simulink model "px4_direct_control"  (R2022b)
settings: Solver=FixedStepAuto  StartTime=0.0  StopTime=inf  RelTol=1e-3
undefined symbols (not defined in the file or in its folder): actuator, timestamp, timestamp_sample, xyz
libraries: ros2lib x8, aerolibutil x6, robotcorelib x1
settings Model: Creator=beniamino  LastModifiedBy=beniamino
settings OptimizationCC: EnhancedBackFolding=on  PassReuseOutputArgsAs=Individual arguments  ZeroExternalMemoryAtStartup=off  ZeroInternalMemoryAtStartup=off  MaxStackSize=64  OptimizeBlockOrder=speed  DifferentSizesBufferReuse=on  OptimizationCustomize=off  EfficientTunableParamExpr=on
settings DebuggingCC: ParameterTunabilityLossMsg=error
settings HardwareCC: ProdBitPerLong=64  ProdHWDeviceType=Intel->x86-64 (Linux 64)
settings SFSimCC: MATLABDynamicMemAlloc=off
settings RTWCC: Description=Embedded Coder  SystemTargetFile=ert.tlc  HardwareBoard=Robot Operating System 2 (ROS 2)  TLCOptions="-aInlineSetEventsForThisBaseRateFcn=TLC_FALSE -aSuppressMultiTaskScheduler=TLC_FALSE  -aRateBasedStepFcn=0"  TemplateMakefile=ert_default_tmf  Toolchain=Colcon Tools  TargetLang=C++
settings CodeAppCC: ForceParamTrailComments=on  IgnoreCustomStorageClasses=off  OperatorAnnotations=on  SimulinkDataObjDesc=on  SFDataObjDesc=on  InsertBlockDesc=on
settings ERTTargetCC: CodeInterfacePackaging=C++ class  RootIOFormat=Structure reference

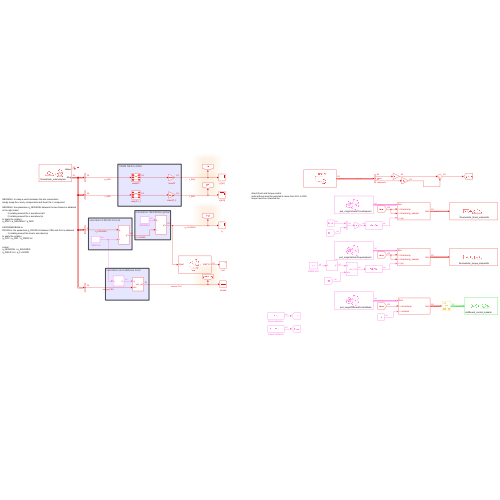
[thumbnail: Simulink's stored preview of the top-level diagram]
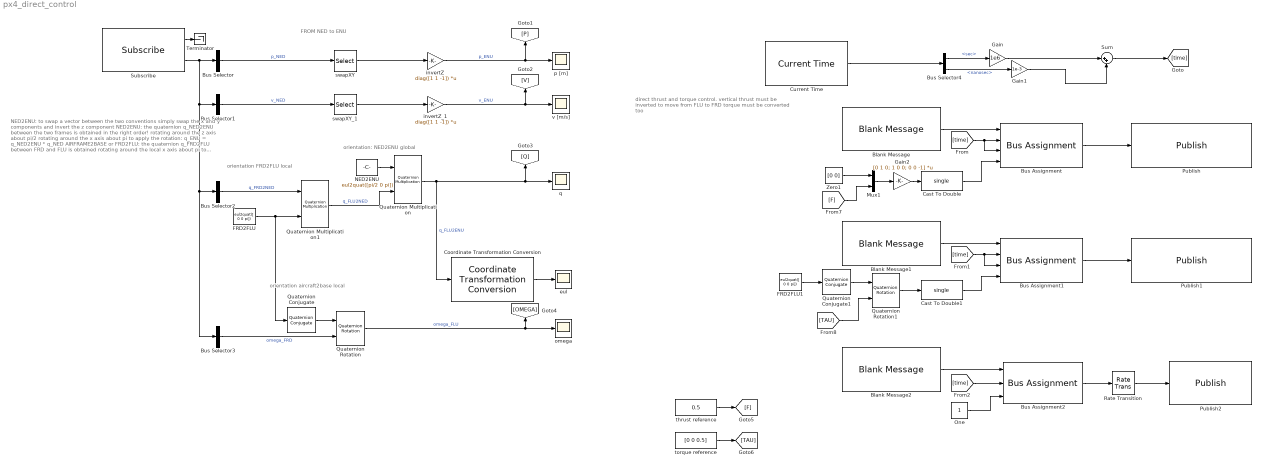
== system px4_direct_control ==
  note: direct thrust and torque control.
      | vertical thrust must be inverted to move from FLU to FRD
      | torque must be converted too
  note: orientation FRD2FLU local
  note: orientation: NED2ENU global
  note: FROM NED to ENU
  note: orientation aircraft2base local
  note: NED2ENU: to swap a vector between the two conventions
      | simply swap the x and y components and invert the z component
      |
      | NED2ENU: the quaternion q_NED2ENU between the two frames is obtained
      | in the right order!
      | rotating around the z axis about pi/2
      | rotating around the x axis about pi
      | to apply the rotation:
      | q_ENU = q_NED2ENU * q_NED
      |
      | AIRFRAME2BASE or
      | FRD2FLU: the quaternion q_FRD2FLU between FRD and FLU is obtained
      | rotating around the local x axis about pi
      | to apply the rotation
      | q_FLU = q_FRD * q_FRD2FLU
      |
      | notice!
      | q_NED2ENU = q_ENU2NED
      | q_FRD2FLU = q_FLU2FRD
  Blank Message : ros2lib/Blank Message  messageClass=Message  entityType=px4_msgs/VehicleThrustSetpoint  messageType=px4_msgs/VehicleThrustSetpoint  SampleTime=inf
      settings: LibrarySourceBlock=roslib/ROS 2/Blank Message
  Blank Message1 : ros2lib/Blank Message  messageClass=Message  entityType=px4_msgs/VehicleTorqueSetpoint  messageType=px4_msgs/VehicleTorqueSetpoint  SampleTime=inf
      settings: LibrarySourceBlock=roslib/ROS 2/Blank Message
  Blank Message2 : ros2lib/Blank Message  messageClass=Message  entityType=px4_msgs/OffboardControlMode  messageType=px4_msgs/OffboardControlMode  SampleTime=inf
      settings: LibrarySourceBlock=roslib/ROS 2/Blank Message
  Bus Assignment : BusAssignment  AssignedSignals=timestamp,timestamp_sample,xyz
  Bus Assignment1 : BusAssignment  AssignedSignals=timestamp,timestamp_sample,xyz
  Bus Assignment2 : BusAssignment  AssignedSignals=timestamp,actuator
  Bus Selector : BusSelector  OutputSignals=position  OutputAsBus=on
  Bus Selector1 : BusSelector  OutputSignals=velocity  OutputAsBus=on
  Bus Selector2 : BusSelector  OutputSignals=q  OutputAsBus=on
  Bus Selector3 : BusSelector  OutputSignals=angular_velocity  OutputAsBus=on
  Bus Selector4 : BusSelector  OutputSignals=sec,nanosec
  Cast To Double : DataTypeConversion  OutDataTypeStr=single  SaturateOnIntegerOverflow=off  RndMeth=Floor
  Cast To Double1 : DataTypeConversion  OutDataTypeStr=single  SaturateOnIntegerOverflow=off  RndMeth=Floor
  Coordinate Transformation Conversion : robotcorelib/Coordinate Transformation Conversion  InputRepresentation=Quaternion  InputEulerSequence=ZYX  ShowTrVecInputPort=on  OutputRepresentation=Euler Angles  OutputEulerSequence=ZYX  ShowTrVecOutputPort=on  SimulateUsing=Code generation
      settings: LibrarySourceBlock=roslib/Utilities/Coordinate Transformation Conversion
  Current Time : ros2lib/Current Time  OutputFormat=bus  SampleTime=0.01  ModelName=px4_tests
      settings: LibrarySourceBlock=roslib/ROS 2/Current Time
  FRD2FLU : Constant  Value=eul2quat([ 0 0 pi])  OutDataTypeStr=single
  FRD2FLU1 : Constant  Value=eul2quat([ 0 0 pi])
  Gain : Gain  Gain=1e6  OutDataTypeStr=double
  Gain1 : Gain  Gain=1e-3  OutDataTypeStr=double
  Gain2 : Gain  Gain=[0 1 0; 1 0 0; 0 0 -1]  Multiplication=Matrix(K*u) (u vector)
  Mux1 : Mux  Inputs=2
  NED2ENU : Constant  Value=eul2quat([pi/2 0 pi])  OutDataTypeStr=single
  One : Constant  OutDataTypeStr=boolean
  Publish : ros2lib/Publish  topicSource=Select from ROS network  topic=/fmu/vehicle_thrust_setpoint/in  messageType=px4_msgs/VehicleThrustSetpoint  QOSHistory=Keep last  QOSDepth=1  QOSReliability=Best effort  QOSDurability=Volatile
      settings: LibrarySourceBlock=roslib/ROS 2/Publish
  Publish1 : ros2lib/Publish  topicSource=Select from ROS network  topic=/fmu/vehicle_torque_setpoint/in  messageType=px4_msgs/VehicleTorqueSetpoint  QOSHistory=Keep last  QOSDepth=1  QOSReliability=Best effort  QOSDurability=Volatile
      settings: LibrarySourceBlock=roslib/ROS 2/Publish
  Publish2 : ros2lib/Publish  topicSource=Select from ROS network  topic=/fmu/offboard_control_mode/in  messageType=px4_msgs/OffboardControlMode  QOSHistory=Keep last  QOSDepth=1  QOSReliability=Best effort  QOSDurability=Volatile
      settings: LibrarySourceBlock=roslib/ROS 2/Publish
  Quaternion Conjugate : aerolibutil/Quaternion Conjugate
  Quaternion Conjugate1 : aerolibutil/Quaternion Conjugate
  Quaternion Multiplication : aerolibutil/Quaternion Multiplication
  Quaternion Multiplication1 : aerolibutil/Quaternion Multiplication
  Quaternion Rotation : aerolibutil/Quaternion Rotation
  Quaternion Rotation1 : aerolibutil/Quaternion Rotation
  Rate Transition : RateTransition  OutPortSampleTime=0.1
  Subscribe : ros2lib/Subscribe  topicSource=Select from ROS network  topic=/fmu/vehicle_odometry/out  messageType=px4_msgs/VehicleOdometry  sampleTime=0.01  QOSHistory=Keep last  QOSDepth=1  QOSReliability=Reliable  QOSDurability=Volatile
      settings: LibrarySourceBlock=roslib/ROS 2/Subscribe
  Sum : Sum  Inputs=|++
  Terminator : Terminator
  Zero1 : Constant  Value=[0 0]  OutDataTypeStr=Inherit: Inherit via back propagation
  eul : Scope
  invertZ : Gain  Gain=diag([1 1 -1])  Multiplication=Matrix(K*u) (u vector)
  invertZ_1 : Gain  Gain=diag([1 1 -1])  Multiplication=Matrix(K*u) (u vector)
  omega : Scope
  p [m] : Scope
  q : Scope
  swapXY : Selector  InputPortWidth=3  IndexOptions=Index vector (dialog)  Indices=[2 1 3]  OutputSizes=1
  swapXY_1 : Selector  InputPortWidth=3  IndexOptions=Index vector (dialog)  Indices=[2 1 3]  OutputSizes=1
  thrust reference : Constant  Value=0.5
  torque reference : Constant  Value=[0 0 0.5]
  v [m/s] : Scope
  wires:
  Subscribe/2 -> Bus Selector1/1, Bus Selector3/1, Bus Selector2/1, Bus Selector/1
  Bus Selector/1 -> swapXY/1  "p_NED"
  invertZ/1 -> p [m]/1, [P]  "p_ENU"
  swapXY/1 -> invertZ/1
  Bus Selector1/1 -> swapXY_1/1  "v_NED"
  swapXY_1/1 -> invertZ_1/1
  invertZ_1/1 -> [V], v [m/s]/1  "v_ENU"
  Bus Selector2/1 -> Quaternion Multiplication1/1  "q_FRD2NED"
  Quaternion Multiplication/1 -> Coordinate Transformation Conversion/1, [Q], q/1  "q_FLU2ENU"
  NED2ENU/1 -> Quaternion Multiplication/1
  Subscribe/1 -> Terminator/1
  Quaternion Multiplication1/1 -> Quaternion Multiplication/2  "q_FLU2NED"
  FRD2FLU/1 -> Quaternion Conjugate/1, Quaternion Multiplication1/2
  Coordinate Transformation Conversion/1 -> eul/1
  Bus Selector3/1 -> Quaternion Rotation/2  "omega_FRD"
  Quaternion Conjugate/1 -> Quaternion Rotation/1
  Quaternion Rotation/1 -> [OMEGA], omega/1  "omega_FLU"
  Blank Message/1 -> Bus Assignment/1
  Blank Message1/1 -> Bus Assignment1/1
  Current Time/1 -> Bus Selector4/1
  Bus Selector4/1 -> Gain/1  "<sec>"
  Gain/1 -> Sum/1
  Bus Selector4/2 -> Gain1/1  "<nanosec>"
  Gain1/1 -> Sum/2
  Sum/1 -> [time]
  [time] -> Bus Assignment/3, Bus Assignment/2
  [time] -> Bus Assignment1/3, Bus Assignment1/2
  [F] -> Mux1/2
  [TAU] -> Quaternion Rotation1/2
  Bus Assignment/1 -> Publish/1
  Bus Assignment1/1 -> Publish1/1
  Blank Message2/1 -> Bus Assignment2/1
  [time] -> Bus Assignment2/2
  One/1 -> Bus Assignment2/3
  Bus Assignment2/1 -> Rate Transition/1
  Rate Transition/1 -> Publish2/1
  Quaternion Conjugate1/1 -> Quaternion Rotation1/1
  FRD2FLU1/1 -> Quaternion Conjugate1/1
  Cast To Double1/1 -> Bus Assignment1/4
  Gain2/1 -> Cast To Double/1
  Cast To Double/1 -> Bus Assignment/4
  Quaternion Rotation1/1 -> Cast To Double1/1
  Mux1/1 -> Gain2/1
  Zero1/1 -> Mux1/1
  thrust reference/1 -> [F]
  torque reference/1 -> [TAU]
